simulink model "MicroFSMPCCLACPU1"  (R2024a)
settings: Solver=FixedStepAuto  StartTime=0.0  StopTime=Inf  RelTol=1e-3  EnableMultiTasking=on
values from neighbouring files (symbols this model uses):
  ar = single(round(1/10,3))    [Para_Motor_Micro.m]
  PI_params = mcb.internal.SetControllerParameters(pmsm,inverter,SI_System,T_pwm,Ts,Ts_speed)    [Para_Motor_Micro.m]
  Tabf = round(Tab',3)    [Para_Motor_Micro.m]
  target = mcb_SetProcessorDetails('F28379D',PWM_frequency)    [Para_Motor_Micro.m]
  Ts = T_pwm    (= 3e-05)    [Para_Motor_Micro.m]
  Ts_com = 2*1*Ts    (= 6e-05)    [Para_Motor_Micro.m]
undefined symbols (not defined in the file or in its folder): C28x, codertarget, CPU1, CPU2, Down, dyV, gmax, GPTRIP1SEL, GPTRIP2SEL, inverter, Ls, PWM_Counter_PeriodVel, R, Tab, Tv, Tvz, TZ1, TZ2, ud, Up
libraries: mcbcontrolslib x28, c2802xlib x18, c2837xDlib x13, dsparch4 x6, eeTransforms x5, slpidlib x4, mcbpositiondecoderlib x3, simulink x2, c2806xlib x1, spsabctoAlphaBetaZeroLib x1, c280xlib x1, c2000lib x1
(part 4 of 8)

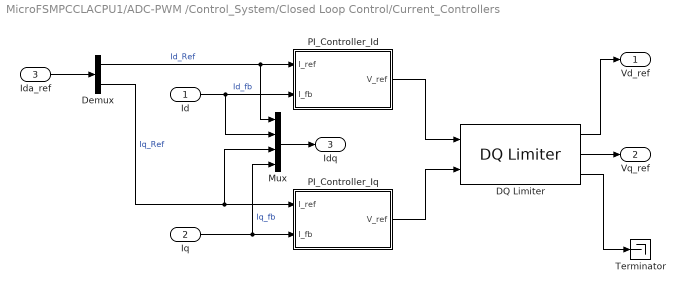
== system MicroFSMPCCLACPU1/ADC-PWM /Control_System/Closed Loop Control/Current_Controllers ==
  Id : Inport
  Iq : Inport  Port=2
  Ida_ref : Inport  Port=3
  DQ Limiter : mcbcontrolslib/DQ Limiter  satMethodInputType=Specify via dialog  satMethodSelected=D-Q equivalence  satLimitInputType=Specify via dialog  Vmax=inverter.V_dc/sqrt(3) *0.95
  Demux : Demux  Outputs=2
  Mux : Mux
  PI_Controller_Id : Subsystem
  PI_Controller_Iq : Subsystem
  Terminator : Terminator
  Vd_ref : Outport  VectorParamsAs1DForOutWhenUnconnected=off
  Vq_ref : Outport  Port=2  VectorParamsAs1DForOutWhenUnconnected=off
  Idq : Outport  Port=3  VectorParamsAs1DForOutWhenUnconnected=off
  wires:
  Iq/1 -> Mux/4, PI_Controller_Iq/2(I_fb)  "Iq_fb"
  Id/1 -> Mux/2, PI_Controller_Id/2(I_fb)  "Id_fb"
  Demux/1 -> Mux/1, PI_Controller_Id/1(I_ref)  "Id_Ref"
  Demux/2 -> Mux/3, PI_Controller_Iq/1(I_ref)  "Iq_Ref"
  Ida_ref/1 -> Demux/1
  Mux/1 -> Idq/1
  PI_Controller_Id/1(V_ref) -> DQ Limiter/1
  PI_Controller_Iq/1(V_ref) -> DQ Limiter/2
  DQ Limiter/2 -> Vq_ref/1
  DQ Limiter/1 -> Vd_ref/1
  DQ Limiter/3 -> Terminator/1

== system MicroFSMPCCLACPU1/ADC-PWM /Control_System/Closed Loop Control/Subsystem ==
  FCEM : Inport
  Demux5 : Demux  Outputs=2
  IIR Filter10 : mcbcontrolslib/IIR Filter  VariantControl=Low Pass Filter  VariantSelect=Low-pass  Filter_constant=0.2  advancedSettings=off  Ts=5e-5  cutOff_freq=795.7747
  IIR Filter9 : mcbcontrolslib/IIR Filter  VariantControl=Low Pass Filter  VariantSelect=Low-pass  Filter_constant=0.2  advancedSettings=off  Ts=5e-5  cutOff_freq=795.7747
  Mux7 : Mux  Inputs=2
  Out1 : Outport
  wires:
  IIR Filter9/1 -> Mux7/1
  Demux5/1 -> IIR Filter9/1
  Demux5/2 -> IIR Filter10/1
  IIR Filter10/1 -> Mux7/2
  Mux7/1 -> Out1/1
  FCEM/1 -> Demux5/1

== system MicroFSMPCCLACPU1/ADC-PWM /Mesurments/Position Mesurment/IndexFinder ==
  In1 : Inport
  Enable : EnablePort
  AND : Logic  AllPortsSameDT=off  OutDataTypeStr=boolean
  Compare To Constant : simulink/Logic and Bit Operations/Compare To Constant  relop===  const=0  OutDataTypeStr=boolean
  Compare To Constant1 : simulink/Logic and Bit Operations/Compare To Constant  relop=>  const=0  OutDataTypeStr=boolean
  Delay3 : Delay  DelayLength=1
  EnClosedLoop : Outport
  wires:
  In1/1 -> Delay3/1, Compare To Constant1/1
  Compare To Constant1/1 -> AND/2
  Compare To Constant/1 -> AND/1
  Delay3/1 -> Compare To Constant/1
  AND/1 -> EnClosedLoop/1

== system MicroFSMPCCLACPU1/ADC-PWM /Control_System/CLA Subsystem Current control/Current_Controllers/PI_Controller_Id ==
  I_ref : Inport
  I_fb : Inport  Port=2
  Data Store Read1 : DataStoreRead  DataStoreName=Enable  IndexOptions=Index vector (dialog)  Indices=1  OutputSizes=1
  Discrete PI Controller with anti-windup & reset : slpidlib/PID Controller  Controller=PI  Form=Parallel  TimeDomain=Discrete-time  UseExternalTs=off  SampleTime=-1  IntegratorMethod=Forward Euler  FilterMethod=Forward Euler  ControllerParametersSource=external  P=1  I=1  UseKiTs=on  D=0  N=100  UseFilter=on  TunerSelectOption=Transfer Function Based (PID Tuner App)  InitialConditionSource=external  InitialConditionForIntegrator=0  InitialConditionForFilter=0  DifferentiatorICPrevScaledInput=0  ExternalReset=level  TrackingMode=off  Kt=1  LimitOutput=on  SatLimitsSource=internal  UpperSaturationLimit=inverter.V_dc/sqrt(3)  LowerSaturationLimit=-inverter.V_dc/sqrt(3)  LinearizeAsGain=on  AntiWindupMode=clamping  Kb=1  LimitIntegrator=off  UpperIntegratorSaturationLimit=inf  LowerIntegratorSaturationLimit=-inf  RndMeth=Simplest  POutMin=[]  POutMax=[]  IOutMin=[]  IOutMax=[]  DOutMin=[]  DOutMax=[]  NOutMin=[]  NOutMax=[]  SumOutMin=[]  SumOutMax=[]  SaturationOutDataTypeStr=Inherit: Inherit via back propagation  SaturationOutMin=[]  SaturationOutMax=[]  PParamMin=[]  PParamMax=[]  IParamMin=[]  IParamMax=[]  DParamMin=[]  DParamMax=[]  NParamMin=[]  NParamMax=[]  KbParamMin=[]  KbParamMax=[]  KtParamMin=[]  KtParamMax=[]  KbOutMin=[]  KbOutMax=[]  KtOutMin=[]  KtOutMax=[]  IntegratorOutMin=[]  IntegratorOutMax=[]  FilterOutMin=[]  FilterOutMax=[]  SumI1OutMin=[]  SumI1OutMax=[]  SumI2OutMin=[]  SumI2OutMax=[]  SumI3OutMin=[]  SumI3OutMax=[]  SumI4OutMin=[]  SumI4OutMax=[]  SumDOutMin=[]  SumDOutMax=[]  DifferentiatorOutMin=[]  DifferentiatorOutMax=[]  FilterDiffOutCoefMin=[]  FilterDiffOutCoefMax=[]  ReciprocalOutMin=[]  ReciprocalOutMax=[]  SumDenOutMin=[]  SumDenOutMax=[]  SumNumOutMin=[]  SumNumOutMax=[]  DivideOutMin=[]  DivideOutMax=[]  UdiffTsProdOutMin=[]  UdiffTsProdOutMax=[]  NTsProdOutMin=[]  NTsProdOutMax=[]  UintegralTsProdOutMin=[]  UintegralTsProdOutMax=[]  UngainTsProdOutMin=[]  UngainTsProdOutMax=[]  ClampingZeroOutDataTypeStr=Inherit: Inherit via back propagation  ClampingZeroOutMin=[]  ClampingZeroOutMax=[]  FilterDenConstantOutDataTypeStr=Inherit: Inherit via back propagation  FilterDenConstantOutMin=[]  FilterDenConstantOutMax=[]  PCopyOutDataTypeStr=Inherit: Inherit via back propagation  PCopyOutMin=[]  PCopyOutMax=[]  NCopyOutDataTypeStr=Inherit: Inherit via back propagation  NCopyOutMin=[]  NCopyOutMax=[]  IntegratorContinuousStateAttributes=''  IntegratorStateMustResolveToSignalObject=off  IntegratorRTWStateStorageClass=Auto  FilterContinuousStateAttributes=''  FilterStateMustResolveToSignalObject=off  FilterRTWStateStorageClass=Auto  ParallelPVariant=ExternalParameters  IdealPVariant=Disabled  IVariant=ExternalParameters  DVariant=Disabled  IntegratorVariant=Discrete  SatVariant=Enabled  AWVariant=DiscClampingParallel  PCopyVariant=Disabled  TRVariant=Disabled  FdbkBlocksVariant=Forward  IdealPFdbkVariant=Disabled  SatFdbkVariant=Disabled  DerivativeFilterVariant=Disabled  NVariant=Disabled  NCopyVariant=Disabled_SignalSpec  FilterICVariant=Disabled  IntegratorICVariant=ExternalICs  ExternalResetVariant=ExternalReset  TRSumVariant=Passthrough  SumFdbkVariant=Disabled  SumVariant=Sum_PI  TsampFilterVariant=InternalTs  TsampNgainVariant=Passthrough  TsampIntegralVariant=Passthrough  ExternalSaturationOutDataTypeStr=Inherit: Same as second input
      settings: LibrarySourceBlock=mcbcontrolslib/PI Controller
  Ki1 : Constant  Value=0  OutDataTypeStr=dataType  SampleTime=-1
  Ki2 : Constant  Value=PI_params.Ki_i * Ts  OutDataTypeStr=dataType  SampleTime=-1
  Kp : Constant  Value=PI_params.Kp_i  OutDataTypeStr=dataType  SampleTime=-1
  Logical Operator : Logic  Operator=NOT  IconShape=distinctive  AllPortsSameDT=off  OutDataTypeStr=boolean
  Sum : Sum  Inputs=|+-  OutDataTypeStr=Inherit: Same as first input
  V_ref : Outport  VectorParamsAs1DForOutWhenUnconnected=off
  wires:
  I_ref/1 -> Sum/1
  I_fb/1 -> Sum/2
  Data Store Read1/1 -> Logical Operator/1
  Discrete PI Controller with anti-windup & reset/1 -> V_ref/1
  Sum/1 -> Discrete PI Controller with anti-windup & reset/1
  Logical Operator/1 -> Discrete PI Controller with anti-windup & reset/4
  Ki1/1 -> Discrete PI Controller with anti-windup & reset/5
  Kp/1 -> Discrete PI Controller with anti-windup & reset/2
  Ki2/1 -> Discrete PI Controller with anti-windup & reset/3

== system MicroFSMPCCLACPU1/ADC-PWM /Control_System/CLA Subsystem Current control/Current_Controllers/PI_Controller_Iq ==
  I_ref : Inport
  I_fb : Inport  Port=2
  Data Store Read1 : DataStoreRead  DataStoreName=Enable  IndexOptions=Index vector (dialog)  Indices=1  OutputSizes=1
  Discrete PI Controller with anti-windup & reset : slpidlib/PID Controller  Controller=PI  Form=Parallel  TimeDomain=Discrete-time  UseExternalTs=off  SampleTime=-1  IntegratorMethod=Forward Euler  FilterMethod=Forward Euler  ControllerParametersSource=external  P=1  I=1  UseKiTs=on  D=0  N=100  UseFilter=on  TunerSelectOption=Transfer Function Based (PID Tuner App)  InitialConditionSource=external  InitialConditionForIntegrator=0  InitialConditionForFilter=0  DifferentiatorICPrevScaledInput=0  ExternalReset=level  TrackingMode=off  Kt=1  LimitOutput=on  SatLimitsSource=internal  UpperSaturationLimit=inverter.V_dc/sqrt(3)  LowerSaturationLimit=-inverter.V_dc/sqrt(3)  LinearizeAsGain=on  AntiWindupMode=clamping  Kb=1  LimitIntegrator=off  UpperIntegratorSaturationLimit=inf  LowerIntegratorSaturationLimit=-inf  RndMeth=Simplest  POutMin=[]  POutMax=[]  IOutMin=[]  IOutMax=[]  DOutMin=[]  DOutMax=[]  NOutMin=[]  NOutMax=[]  SumOutMin=[]  SumOutMax=[]  SaturationOutDataTypeStr=Inherit: Inherit via back propagation  SaturationOutMin=[]  SaturationOutMax=[]  PParamMin=[]  PParamMax=[]  IParamMin=[]  IParamMax=[]  DParamMin=[]  DParamMax=[]  NParamMin=[]  NParamMax=[]  KbParamMin=[]  KbParamMax=[]  KtParamMin=[]  KtParamMax=[]  KbOutMin=[]  KbOutMax=[]  KtOutMin=[]  KtOutMax=[]  IntegratorOutMin=[]  IntegratorOutMax=[]  FilterOutMin=[]  FilterOutMax=[]  SumI1OutMin=[]  SumI1OutMax=[]  SumI2OutMin=[]  SumI2OutMax=[]  SumI3OutMin=[]  SumI3OutMax=[]  SumI4OutMin=[]  SumI4OutMax=[]  SumDOutMin=[]  SumDOutMax=[]  DifferentiatorOutMin=[]  DifferentiatorOutMax=[]  FilterDiffOutCoefMin=[]  FilterDiffOutCoefMax=[]  ReciprocalOutMin=[]  ReciprocalOutMax=[]  SumDenOutMin=[]  SumDenOutMax=[]  SumNumOutMin=[]  SumNumOutMax=[]  DivideOutMin=[]  DivideOutMax=[]  UdiffTsProdOutMin=[]  UdiffTsProdOutMax=[]  NTsProdOutMin=[]  NTsProdOutMax=[]  UintegralTsProdOutMin=[]  UintegralTsProdOutMax=[]  UngainTsProdOutMin=[]  UngainTsProdOutMax=[]  ClampingZeroOutDataTypeStr=Inherit: Inherit via back propagation  ClampingZeroOutMin=[]  ClampingZeroOutMax=[]  FilterDenConstantOutDataTypeStr=Inherit: Inherit via back propagation  FilterDenConstantOutMin=[]  FilterDenConstantOutMax=[]  PCopyOutDataTypeStr=Inherit: Inherit via back propagation  PCopyOutMin=[]  PCopyOutMax=[]  NCopyOutDataTypeStr=Inherit: Inherit via back propagation  NCopyOutMin=[]  NCopyOutMax=[]  IntegratorContinuousStateAttributes=''  IntegratorStateMustResolveToSignalObject=off  IntegratorRTWStateStorageClass=Auto  FilterContinuousStateAttributes=''  FilterStateMustResolveToSignalObject=off  FilterRTWStateStorageClass=Auto  ParallelPVariant=ExternalParameters  IdealPVariant=Disabled  IVariant=ExternalParameters  DVariant=Disabled  IntegratorVariant=Discrete  SatVariant=Enabled  AWVariant=DiscClampingParallel  PCopyVariant=Disabled  TRVariant=Disabled  FdbkBlocksVariant=Forward  IdealPFdbkVariant=Disabled  SatFdbkVariant=Disabled  DerivativeFilterVariant=Disabled  NVariant=Disabled  NCopyVariant=Disabled_SignalSpec  FilterICVariant=Disabled  IntegratorICVariant=ExternalICs  ExternalResetVariant=ExternalReset  TRSumVariant=Passthrough  SumFdbkVariant=Disabled  SumVariant=Sum_PI  TsampFilterVariant=InternalTs  TsampNgainVariant=Passthrough  TsampIntegralVariant=Passthrough  ExternalSaturationOutDataTypeStr=Inherit: Same as second input
      settings: LibrarySourceBlock=mcbcontrolslib/PI Controller
  Ki1 : Constant  Value=PI_params.Ki_i * Ts  OutDataTypeStr=dataType  SampleTime=-1
  Kp : Constant  Value=PI_params.Kp_i  OutDataTypeStr=dataType  SampleTime=-1
  Kp1 : Constant  Value=0  OutDataTypeStr=dataType  SampleTime=-1
  Logical Operator : Logic  Operator=NOT  IconShape=distinctive  AllPortsSameDT=off  OutDataTypeStr=boolean
  Sum : Sum  Inputs=|+-  OutDataTypeStr=Inherit: Same as first input
  V_ref : Outport  VectorParamsAs1DForOutWhenUnconnected=off
  wires:
  Discrete PI Controller with anti-windup & reset/1 -> V_ref/1
  Data Store Read1/1 -> Logical Operator/1
  I_fb/1 -> Sum/2
  I_ref/1 -> Sum/1
  Sum/1 -> Discrete PI Controller with anti-windup & reset/1
  Logical Operator/1 -> Discrete PI Controller with anti-windup & reset/4
  Kp1/1 -> Discrete PI Controller with anti-windup & reset/5
  Kp/1 -> Discrete PI Controller with anti-windup & reset/2
  Ki1/1 -> Discrete PI Controller with anti-windup & reset/3

== system MicroFSMPCCLACPU1/ADC-PWM /Control_System/Closed Loop Control/Current_Controllers/PI_Controller_Id ==
  I_ref : Inport
  I_fb : Inport  Port=2
  Data Store Read1 : DataStoreRead  DataStoreName=Enable  IndexOptions=Index vector (dialog)  Indices=1  OutputSizes=1
  Discrete PI Controller with anti-windup & reset : slpidlib/PID Controller  Controller=PI  Form=Parallel  TimeDomain=Discrete-time  UseExternalTs=off  SampleTime=-1  IntegratorMethod=Forward Euler  FilterMethod=Forward Euler  ControllerParametersSource=external  P=1  I=1  UseKiTs=on  D=0  N=100  UseFilter=on  TunerSelectOption=Transfer Function Based (PID Tuner App)  InitialConditionSource=external  InitialConditionForIntegrator=0  InitialConditionForFilter=0  DifferentiatorICPrevScaledInput=0  ExternalReset=level  TrackingMode=off  Kt=1  LimitOutput=on  SatLimitsSource=internal  UpperSaturationLimit=inverter.V_dc/sqrt(3)  LowerSaturationLimit=-inverter.V_dc/sqrt(3)  LinearizeAsGain=on  AntiWindupMode=clamping  Kb=1  LimitIntegrator=off  UpperIntegratorSaturationLimit=inf  LowerIntegratorSaturationLimit=-inf  RndMeth=Simplest  POutMin=[]  POutMax=[]  IOutMin=[]  IOutMax=[]  DOutMin=[]  DOutMax=[]  NOutMin=[]  NOutMax=[]  SumOutMin=[]  SumOutMax=[]  SaturationOutDataTypeStr=Inherit: Inherit via back propagation  SaturationOutMin=[]  SaturationOutMax=[]  PParamMin=[]  PParamMax=[]  IParamMin=[]  IParamMax=[]  DParamMin=[]  DParamMax=[]  NParamMin=[]  NParamMax=[]  KbParamMin=[]  KbParamMax=[]  KtParamMin=[]  KtParamMax=[]  KbOutMin=[]  KbOutMax=[]  KtOutMin=[]  KtOutMax=[]  IntegratorOutMin=[]  IntegratorOutMax=[]  FilterOutMin=[]  FilterOutMax=[]  SumI1OutMin=[]  SumI1OutMax=[]  SumI2OutMin=[]  SumI2OutMax=[]  SumI3OutMin=[]  SumI3OutMax=[]  SumI4OutMin=[]  SumI4OutMax=[]  SumDOutMin=[]  SumDOutMax=[]  DifferentiatorOutMin=[]  DifferentiatorOutMax=[]  FilterDiffOutCoefMin=[]  FilterDiffOutCoefMax=[]  ReciprocalOutMin=[]  ReciprocalOutMax=[]  SumDenOutMin=[]  SumDenOutMax=[]  SumNumOutMin=[]  SumNumOutMax=[]  DivideOutMin=[]  DivideOutMax=[]  UdiffTsProdOutMin=[]  UdiffTsProdOutMax=[]  NTsProdOutMin=[]  NTsProdOutMax=[]  UintegralTsProdOutMin=[]  UintegralTsProdOutMax=[]  UngainTsProdOutMin=[]  UngainTsProdOutMax=[]  ClampingZeroOutDataTypeStr=Inherit: Inherit via back propagation  ClampingZeroOutMin=[]  ClampingZeroOutMax=[]  FilterDenConstantOutDataTypeStr=Inherit: Inherit via back propagation  FilterDenConstantOutMin=[]  FilterDenConstantOutMax=[]  PCopyOutDataTypeStr=Inherit: Inherit via back propagation  PCopyOutMin=[]  PCopyOutMax=[]  NCopyOutDataTypeStr=Inherit: Inherit via back propagation  NCopyOutMin=[]  NCopyOutMax=[]  IntegratorContinuousStateAttributes=''  IntegratorStateMustResolveToSignalObject=off  IntegratorRTWStateStorageClass=Auto  FilterContinuousStateAttributes=''  FilterStateMustResolveToSignalObject=off  FilterRTWStateStorageClass=Auto  ParallelPVariant=ExternalParameters  IdealPVariant=Disabled  IVariant=ExternalParameters  DVariant=Disabled  IntegratorVariant=Discrete  SatVariant=Enabled  AWVariant=DiscClampingParallel  PCopyVariant=Disabled  TRVariant=Disabled  FdbkBlocksVariant=Forward  IdealPFdbkVariant=Disabled  SatFdbkVariant=Disabled  DerivativeFilterVariant=Disabled  NVariant=Disabled  NCopyVariant=Disabled_SignalSpec  FilterICVariant=Disabled  IntegratorICVariant=ExternalICs  ExternalResetVariant=ExternalReset  TRSumVariant=Passthrough  SumFdbkVariant=Disabled  SumVariant=Sum_PI  TsampFilterVariant=InternalTs  TsampNgainVariant=Passthrough  TsampIntegralVariant=Passthrough  ExternalSaturationOutDataTypeStr=Inherit: Same as second input
      settings: LibrarySourceBlock=mcbcontrolslib/PI Controller
  Ki1 : Constant  Value=0  OutDataTypeStr=dataType  SampleTime=-1
  Ki2 : Constant  Value=PI_params.Ki_i * Ts  OutDataTypeStr=dataType  SampleTime=-1
  Kp : Constant  Value=PI_params.Kp_i  OutDataTypeStr=dataType  SampleTime=-1
  Logical Operator : Logic  Operator=NOT  IconShape=distinctive  AllPortsSameDT=off  OutDataTypeStr=boolean
  Sum : Sum  Inputs=|+-  OutDataTypeStr=Inherit: Same as first input
  V_ref : Outport  VectorParamsAs1DForOutWhenUnconnected=off
  wires:
  I_ref/1 -> Sum/1
  I_fb/1 -> Sum/2
  Data Store Read1/1 -> Logical Operator/1
  Discrete PI Controller with anti-windup & reset/1 -> V_ref/1
  Sum/1 -> Discrete PI Controller with anti-windup & reset/1
  Logical Operator/1 -> Discrete PI Controller with anti-windup & reset/4
  Ki1/1 -> Discrete PI Controller with anti-windup & reset/5
  Kp/1 -> Discrete PI Controller with anti-windup & reset/2
  Ki2/1 -> Discrete PI Controller with anti-windup & reset/3

== system MicroFSMPCCLACPU1/ADC-PWM /Control_System/Closed Loop Control/Current_Controllers/PI_Controller_Iq ==
  I_ref : Inport
  I_fb : Inport  Port=2
  Data Store Read1 : DataStoreRead  DataStoreName=Enable  IndexOptions=Index vector (dialog)  Indices=1  OutputSizes=1
  Discrete PI Controller with anti-windup & reset : slpidlib/PID Controller  Controller=PI  Form=Parallel  TimeDomain=Discrete-time  UseExternalTs=off  SampleTime=-1  IntegratorMethod=Forward Euler  FilterMethod=Forward Euler  ControllerParametersSource=external  P=1  I=1  UseKiTs=on  D=0  N=100  UseFilter=on  TunerSelectOption=Transfer Function Based (PID Tuner App)  InitialConditionSource=external  InitialConditionForIntegrator=0  InitialConditionForFilter=0  DifferentiatorICPrevScaledInput=0  ExternalReset=level  TrackingMode=off  Kt=1  LimitOutput=on  SatLimitsSource=internal  UpperSaturationLimit=inverter.V_dc/sqrt(3)  LowerSaturationLimit=-inverter.V_dc/sqrt(3)  LinearizeAsGain=on  AntiWindupMode=clamping  Kb=1  LimitIntegrator=off  UpperIntegratorSaturationLimit=inf  LowerIntegratorSaturationLimit=-inf  RndMeth=Simplest  POutMin=[]  POutMax=[]  IOutMin=[]  IOutMax=[]  DOutMin=[]  DOutMax=[]  NOutMin=[]  NOutMax=[]  SumOutMin=[]  SumOutMax=[]  SaturationOutDataTypeStr=Inherit: Inherit via back propagation  SaturationOutMin=[]  SaturationOutMax=[]  PParamMin=[]  PParamMax=[]  IParamMin=[]  IParamMax=[]  DParamMin=[]  DParamMax=[]  NParamMin=[]  NParamMax=[]  KbParamMin=[]  KbParamMax=[]  KtParamMin=[]  KtParamMax=[]  KbOutMin=[]  KbOutMax=[]  KtOutMin=[]  KtOutMax=[]  IntegratorOutMin=[]  IntegratorOutMax=[]  FilterOutMin=[]  FilterOutMax=[]  SumI1OutMin=[]  SumI1OutMax=[]  SumI2OutMin=[]  SumI2OutMax=[]  SumI3OutMin=[]  SumI3OutMax=[]  SumI4OutMin=[]  SumI4OutMax=[]  SumDOutMin=[]  SumDOutMax=[]  DifferentiatorOutMin=[]  DifferentiatorOutMax=[]  FilterDiffOutCoefMin=[]  FilterDiffOutCoefMax=[]  ReciprocalOutMin=[]  ReciprocalOutMax=[]  SumDenOutMin=[]  SumDenOutMax=[]  SumNumOutMin=[]  SumNumOutMax=[]  DivideOutMin=[]  DivideOutMax=[]  UdiffTsProdOutMin=[]  UdiffTsProdOutMax=[]  NTsProdOutMin=[]  NTsProdOutMax=[]  UintegralTsProdOutMin=[]  UintegralTsProdOutMax=[]  UngainTsProdOutMin=[]  UngainTsProdOutMax=[]  ClampingZeroOutDataTypeStr=Inherit: Inherit via back propagation  ClampingZeroOutMin=[]  ClampingZeroOutMax=[]  FilterDenConstantOutDataTypeStr=Inherit: Inherit via back propagation  FilterDenConstantOutMin=[]  FilterDenConstantOutMax=[]  PCopyOutDataTypeStr=Inherit: Inherit via back propagation  PCopyOutMin=[]  PCopyOutMax=[]  NCopyOutDataTypeStr=Inherit: Inherit via back propagation  NCopyOutMin=[]  NCopyOutMax=[]  IntegratorContinuousStateAttributes=''  IntegratorStateMustResolveToSignalObject=off  IntegratorRTWStateStorageClass=Auto  FilterContinuousStateAttributes=''  FilterStateMustResolveToSignalObject=off  FilterRTWStateStorageClass=Auto  ParallelPVariant=ExternalParameters  IdealPVariant=Disabled  IVariant=ExternalParameters  DVariant=Disabled  IntegratorVariant=Discrete  SatVariant=Enabled  AWVariant=DiscClampingParallel  PCopyVariant=Disabled  TRVariant=Disabled  FdbkBlocksVariant=Forward  IdealPFdbkVariant=Disabled  SatFdbkVariant=Disabled  DerivativeFilterVariant=Disabled  NVariant=Disabled  NCopyVariant=Disabled_SignalSpec  FilterICVariant=Disabled  IntegratorICVariant=ExternalICs  ExternalResetVariant=ExternalReset  TRSumVariant=Passthrough  SumFdbkVariant=Disabled  SumVariant=Sum_PI  TsampFilterVariant=InternalTs  TsampNgainVariant=Passthrough  TsampIntegralVariant=Passthrough  ExternalSaturationOutDataTypeStr=Inherit: Same as second input
      settings: LibrarySourceBlock=mcbcontrolslib/PI Controller
  Ki1 : Constant  Value=PI_params.Ki_i * Ts  OutDataTypeStr=dataType  SampleTime=-1
  Kp : Constant  Value=PI_params.Kp_i  OutDataTypeStr=dataType  SampleTime=-1
  Kp1 : Constant  Value=0  OutDataTypeStr=dataType  SampleTime=-1
  Logical Operator : Logic  Operator=NOT  IconShape=distinctive  AllPortsSameDT=off  OutDataTypeStr=boolean
  Sum : Sum  Inputs=|+-  OutDataTypeStr=Inherit: Same as first input
  V_ref : Outport  VectorParamsAs1DForOutWhenUnconnected=off
  wires:
  Discrete PI Controller with anti-windup & reset/1 -> V_ref/1
  Data Store Read1/1 -> Logical Operator/1
  I_fb/1 -> Sum/2
  I_ref/1 -> Sum/1
  Sum/1 -> Discrete PI Controller with anti-windup & reset/1
  Logical Operator/1 -> Discrete PI Controller with anti-windup & reset/4
  Kp1/1 -> Discrete PI Controller with anti-windup & reset/5
  Kp/1 -> Discrete PI Controller with anti-windup & reset/2
  Ki1/1 -> Discrete PI Controller with anti-windup & reset/3

== matlab function MicroFSMPCCLACPU1/ADC-PWM /Control_System/CLA Subsystem Current control/TESTCLA ==
  settings: updateMethod=DISCRETE
  data: I input; Gate output size=3; FEM input size=2; moder input single

function Gate       = fcn(I,FEM,moder)
TA=single(0);
TB=single(0);
TC=single(0);
%  persistent    Gates
%      if isempty(Gates)
%         Gates=single([0,0,0]');
%  
%        end

%%%%%%Read mesurments%%%%%%%%%%%%
iA=I(1);
iB=I(2);
eA=FEM(1);
eB=FEM(2);

Ta=single(0.1*0.25);
Tb=single(0.1*0);

TA=single((moder==1)*(Tb+Ta)+(moder==6)*(Tb+Ta)+(moder==2)*(Ta)+(moder==5)*(Tb));
TB=single((moder==1)*(Tb)+(moder==2)*(Tb+Ta)+(moder==3)*(Tb+Ta)+(moder==4)*(Ta));
TC=single((moder==6)*(Ta)+(moder==3)*(Tb)+(moder==4)*(Tb+Ta)+(moder==5)*(Tb+Ta));
  
% TA=single(0.1*moder);
% TB=single(0.1);
% TC=single(0.1);
%%%Optimized modulation.
% if moder==1
% TA=single(Tb+Ta);
% TB=single(Tb);
% TC=single(0);
% elseif moder==2
% TA=single(Ta);
% TB=single(Tb+Ta);
% TC=single(0);
% elseif moder==3
% TA=single(0);
% TB=single(Tb+Ta);
% TC=single(Tb);   
% elseif moder==4
% TA=single(0);
% TB=single(Ta);
% TC=single(Tb+Ta); 
% elseif moder==5
% TA=single(Tb);
% TB=single(0);
% TC=single(Tb+Ta); 
% elseif moder==6
% TA=single(Tb+Ta);
% TB=single(0);
% TC=single(Ta); 
% else
% TA=single(0);
% TB=single(0);
% TC=single(0);   
% end



Gates=[TA,TB,TC]';
Gate=Gates;

== matlab function MicroFSMPCCLACPU1/ADC-PWM /Control_System/CLA Subsystem Current control/FS-MPC opt tiempo complex Clean CLA ==
  settings: updateMethod=DISCRETE
  data: I input single size=2; Gate output single size=3; FEM input single size=2; iAref input single size=1; iBref input single size=1; mode input single size=1; ud input

function Gate       = fcn(I,FEM,iAref,iBref,mode,ud)


%%%%%Init Parameters%%%%%%%
% 
Ts=single(3e-5);
R=single(1) ;
Ls=single(0.002871);
%ud=single(170);
gmax=single(1000);
n=single(11);
moder=mode;
%Tabfn=single([0,0;0,0;0,0;0,0]);
p1=single(0);
p2=single(0);

 persistent     Gates Gop jop  Tr Tao Tbo  
  if isempty(Gates)
        Gates=single([0,0,0]');
        Gop=gmax;
        jop=single(1);
        Tr=single(0);
        Tao=single(0);
Tbo=single(0);

     end


% ar=single(0.9*0.143);
% Tabf=single(0.9*[0.286	0;
% 0	0.286;
% 0.572	0;
% 0	0.572;
% 0.858	0;
% 0	0.858;
% 1	0;
% 0	1;
% 1	0;
% 0	1;
% 0	0;]);

ar=single(0.129);

Tabf=single([0.242	0;
0	0.242;
0.484	0;
0	0.484;
0.726	0;
0	0.726;
1	0;
0	1;
1	0;
0	1;
0	0;]);


%%%%%%Read mesurments%%%%%%%%%%%%
iA=I(1);
iB=I(2);
eA=-FEM(1);
eB=-FEM(2);




% % %%%7 Vectores totales
 if mode==1
 u1=ud*[2/3	,	0	;
1/3	,	1/sqrt(3);
0	,	0	;];
elseif mode==2
 u1=ud*[1/3	,	1/sqrt(3)	;
-1/3	,	1/sqrt(3)	;
0	,	0	;];   
elseif mode==3
 u1=ud*[-1/3	,	1/sqrt(3)	;
-2/3	,	0	;
0	,	0	;];  
 elseif mode==4
 u1=ud*[-2/3	,	0	;
-1/3	,	-1/sqrt(3)	;
0	,	0	;];
 elseif mode==5
 u1=ud*[-1/3	,	-1/sqrt(3)	;
1/3	,	-1/sqrt(3)	;
0	,	0	;];
 elseif mode==6
 u1=ud*[1/3	,	-1/sqrt(3)	;
2/3	,	0	;
0	,	0	;];
else
 u1=ud*[2/3	,	0	;
1/3	,	1/sqrt(3);
0	,	0	;]; 
end
%%%%%%%




%%%%%%%%FSMPC%%%%%%%%%%%%%%%%%%%%%%%%%%%%%%%%%%%%%

      Gop=gmax;
      jop=single(1);
     %  ar=single(0.9/7);
%%%%%%For n loop N1  %%%%%% 





     uA1=u1(1,1);
     uB1=u1(1,2);
     uA2=u1(2,1);
     uB2=u1(2,2);

%%%%%%For n loop  %%%%%% 
     for j= 1:n    
   
if j==7
p1=Tr+ar;
p2=Tr-ar;
end

   if j<=n-5      
    T1=Tabf(j,1);
    T2=Tabf(j,2);
   elseif j<=n-3  
    T1=p1*Tabf(j,1);
    T2=p1*Tabf(j,2);
   else
    T1=p2*Tabf(j,1);
    T2=p2*Tabf(j,2);
   end


   uA=(T1*uA1 + T2*uA2);
   uB=(T1*uB1 + T2*uB2);
     
%%%%%%For loop %%%%%%%%%%%%%%%%%%%%%%%%%%%%%%%%% 
     iA1= iA + (1/Ls)*(Ts*uA)- (Ts/Ls)*(eA+R*iA);
     iB1=iB + (1/Ls)*(Ts*uB)- (Ts/Ls)*(eB+R*iB);

     G=(iAref-iA1)^2+(iBref-iB1)^2 ; 
     % G=abs(iAref-iA1)+abs(iBref-iB1) ; 
          if G<Gop
          Gop=G;
          %jop=j;
          Tr=T1+T2;
          Tao=T1;
          Tbo=T2;
          end
     end
%end
%%%%%%%%%%%%%%%%%%%%%%%%%%%%%%%%%%%%%%%%%%%%%%%%%
    
%%%%Apply conmutation states%%%%%%%%%%%%%%%%%%%%%%%  


Ta=Tao;
Tb=Tbo;
% To=single(1-Ta-Tb-0.1);

TA=(moder==1)*(Tb+Ta)+(moder==6)*(Tb+Ta)+(moder==2)*(Ta)+(moder==5)*(Tb);
TB=(moder==1)*(Tb)+(moder==2)*(Tb+Ta)+(moder==3)*(Tb+Ta)+(moder==4)*(Ta);
TC=(moder==6)*(Ta)+(moder==3)*(Tb)+(moder==4)*(Tb+Ta)+(moder==5)*(Tb+Ta);

% TA=(mode==1)*(To+Tb+Ta)+(mode==6)*(To+Tb+Ta)+(mode==2)*(To+Ta)+(mode==3)*(To)+(mode==4)*(To)+(mode==5)*(To+Tb);
% TB=(mode==6)*(To)+(mode==1)*(To+Tb)+(mode==2)*(To+Tb+Ta)+(mode==3)*(To+Tb+Ta)+(mode==4)*(To+Ta)+(mode==5)*(To);
% TC=(mode==6)*(To+Ta)+(mode==1)*(To)+(mode==2)*(To)+(mode==3)*(To+Tb)+(mode==4)*(To+Tb+Ta)+(mode==5)*(To+Tb+Ta);

Gates=[TA,TB,TC]';
%J=jop;
Gate=Gates;

== matlab function MicroFSMPCCLACPU1/ADC-PWM /Control_System/CLA Subsystem Current control/FS-MPC 2 Vectores solos modulado CLA1 ==
  settings: updateMethod=DISCRETE
  data: I input; Gate output size=3; FEM input size=2; iAref input; iBref input; mode input; ud input

function Gate        = fcn(I,FEM,iAref,iBref,mode,ud)
%function Gate       = fcn(I,FEM,iAref,iBref,mode,Ts, R, Ls, ud, gmax,dyV, Tab)


%%%%%Init Parameters%%%%%%%

Ts=single(4e-5);
R=single(1.1) ;
%Ls=single(0.002871);
Ls=single(0.00372);%%Mediciones
%ud=single(170);
gmax=single(1000);
n=single(15);

% Div=single(4); %%%%Numero de divisiones 
% dy0=single(0.12);
dyV=single(0.85);



%Tp=single(Ts*0.9);
 persistent    Gop jop Gates 
     if isempty(Gates)
        Gates=single([0,0,0]');
        Gop=gmax;
        jop=single(1);
  
     end


%%%%%%Read mesurments%%%%%%%%%%%%
iA=I(1);
iB=I(2);
eA=-FEM(1);
eB=-FEM(2);
moder=mode;

% % 
% % indexv=[1,1,1,1,1,1,1,1,1,1,2,2,2,2,3;
% %         1,1,1,1,1,1,2,2,2,3,2,2,2,3,3;
% %         1,1,1,2,2,3,2,2,3,3,2,2,3,3,3;
% %         1,2,3,2,3,3,2,3,3,3,2,3,3,3,3;];

Tab=single([0.143	0;
0	0.143;
0.286	0;
0	0.286;
0.429	0;
0	0.429;
0.572	0;
0	0.572;
0.715	0;
0	0.715;
0.858	0;
0	0.858;
1	0;
0	1;
0	0]);

if mode==1
   u1=ud*single([0	,	0	;
2/3	,	0	;
1/3	,	1/sqrt(3)]);
elseif mode==2
   u1=ud*single([0	,	0	;
1/3	,	1/sqrt(3)	;
-1/3	,	1/sqrt(3)	;]);   
elseif mode==3
   u1=ud*single([0	,	0	;
-1/3	,	1/sqrt(3)	;
-2/3	,	0	;]);  
 elseif mode==4
   u1=ud*single([0	,	0	;
-2/3	,	0	;
-1/3	,	-1/sqrt(3)	;]);
 elseif mode==5
   u1=ud*single([0	,	0	;
-1/3	,	-1/sqrt(3)	;
1/3	,	-1/sqrt(3)	;]);
 elseif mode==6
  u1=ud*single([0	,	0	;
1/3	,	-1/sqrt(3)	;
2/3	,	0	;]);
else
  u1=ud*single([0	,	0	;
2/3	,	0	;
1/3	,	1/sqrt(3)]); 
end

%%%%%%%%FSMPC%%%%%%%%%%%%%%%%%%%%%%%%%%%%%%%%%%%%%

     Gop=gmax;
     jop=single(1);
     uA1=u1(2,1);
     uB1=u1(2,2);
     uA2=u1(3,1);
     uB2=u1(3,2);

%%%%%%For n loop  %%%%%% 
     for j= 1:n    
   
    T1=Tab(j,1);
    T2=Tab(j,2);
    uA=dyV*(T1*uA1 + T2*uA2);%+dy0*uAnull;
    uB=dyV*(T1*uB1 + T2*uB2);%+dy0*uAnull;

%%%%%%For loop 3 combinacion de vectores%%%%%% 

     iA1= iA + (1/Ls)*(Ts*uA)- (Ts/Ls)*(eA+R*iA);
     iB1=iB + (1/Ls)*(Ts*uB)- (Ts/Ls)*(eB+R*iB);
     
     G=(iAref-iA1)^2+(iBref-iB1)^2 ; 

          if G<Gop
          Gop=G;
          jop=j;
          
          end
     end
%%%%Apply conmutation states%%%%%%%%%%%%%%%%%%%%%%%  
Ta=dyV*Tab(jop,1);
Tb=dyV*Tab(jop,2);
To=1-Ta-Tb-0.15;

% TA=(moder==1)*(Tb+Ta)+(moder==6)*(Tb+Ta)+(moder==2)*(Ta)+(moder==5)*(Tb);
% TB=(moder==1)*(Tb)+(moder==2)*(Tb+Ta)+(moder==3)*(Tb+Ta)+(moder==4)*(Ta);
% TC=(moder==6)*(Ta)+(moder==3)*(Tb)+(moder==4)*(Tb+Ta)+(moder==5)*(Tb+Ta);

TA=(mode==1)*(To+Tb+Ta)+(mode==6)*(To+Tb+Ta)+(mode==2)*(To+Ta)+(mode==3)*(To)+(mode==4)*(To)+(mode==5)*(To+Tb);
TB=(mode==6)*(To)+(mode==1)*(To+Tb)+(mode==2)*(To+Tb+Ta)+(mode==3)*(To+Tb+Ta)+(mode==4)*(To+Ta)+(mode==5)*(To);
TC=(mode==6)*(To+Ta)+(mode==1)*(To)+(mode==2)*(To)+(mode==3)*(To+Tb)+(mode==4)*(To+Tb+Ta)+(mode==5)*(To+Tb+Ta);
  

Gates=[TA,TB,TC]';
Gate=Gates;
%jo=jop;

== matlab function MicroFSMPCCLACPU1/ADC-PWM /Control_System/CLA Subsystem Current control/FS-MPC Simple CLA Mod ==
  settings: updateMethod=DISCRETE
  data: I input; Gate output size=3; FEM input; iAref input; iBref input; mode input; ud input

function Gate       = fcn(I,FEM,iAref,iBref,mode,ud)
%function [Gate,J,Vpred,Ipred]      = fcn(I,FEM,iAref,iBref,Vbus,mode)


%%%%%Init Parameters%%%%%%%
Ts=single(3e-5);
R=single(1.1) ;
%Ls=single(0.002871);
Ls=single(0.00372);%%Mediciones
ud=single(170);
gmax=single(1000);

n=single(3);
Tp=single(Ts*0.85);

 persistent    Gop jop Gates  %status1 %tick status1 
     if isempty(Gates)
        Gates=single([0,0,0]');
        Gop=gmax;
        jop=single(1);
     end


%%%%%%Read mesurments%%%%%%%%%%%%
iA=I(1);
iB=I(2);
eA=-FEM(1);
eB=-FEM(2);
moder=mode;

%%%% 7 vectors
%  status1=single([0,0,0;
%  1,0,0;
%  1,1,0; 
%  0,1,0;
%  0,1,1;
%  0,0,1;
%  1,0,1;]);   
%  u1=ud*single([0	,	0	;
%  2/3	,	0	;
%  1/3	,	1/sqrt(3);
% -1/3	,	1/sqrt(3);
% -2/3	,	0;
% -1/3	,	-1/sqrt(3);
%  1/3	,	-1/sqrt(3)	;]);
%%%%%%%


%%%%% Como en sim 
 if mode==1

 u1=ud*single([0	,	0	;
2/3	,	0	;
1/3	,	1/sqrt(3)]);
elseif mode==2

 u1=ud*single([0	,	0	;
1/3	,	1/sqrt(3)	;
-1/3	,	1/sqrt(3)	;]);   
elseif mode==3

 u1=ud*single([0	,	0	;
-1/3	,	1/sqrt(3)	;
-2/3	,	0	;]);  
 elseif mode==4

 u1=ud*single([0	,	0	;
-2/3	,	0	;
-1/3	,	-1/sqrt(3)	;]);
 elseif mode==5

 u1=ud*single([0	,	0	;
-1/3	,	-1/sqrt(3)	;
1/3	,	-1/sqrt(3)	;]);
 elseif mode==6

 u1=ud*single([0	,	0	;
1/3	,	-1/sqrt(3)	;
2/3	,	0	;]);

else

 u1=ud*single([0	,	0	;
2/3	,	0	;
1/3	,	1/sqrt(3)]); 
end






%%%%%%%%FSMPC%%%%%%%%%%%%%%%%%%%%%%%%%%%%%%%%%%%%%

     Gop=gmax;

%%%%%%For n loop  %%%%%% 
     for j= 1:n    
     uA1=u1(j,1);
     uB1=u1(j,2);


     iA1= iA + (1/Ls)*(Tp*uA1)- (Ts/Ls)*(eA+R*iA);
     iB1=iB + (1/Ls)*(Tp*uB1)- (Ts/Ls)*(eB+R*iB);
     
    
     G=(iAref-iA1)^2+(iBref-iB1)^2;%+ b*Z ; 

          if G<Gop
          Gop=G;
          jop=j;
          end
     end




Ta=single(0.85)*(jop==2);
Tb=single(0.85)*(jop==3);
% 
TA=(moder==1)*(Tb+Ta)+(moder==6)*(Tb+Ta)+(moder==2)*(Ta)+(moder==5)*(Tb);
TB=(moder==1)*(Tb)+(moder==2)*(Tb+Ta)+(moder==3)*(Tb+Ta)+(moder==4)*(Ta);
TC=(moder==6)*(Ta)+(moder==3)*(Tb)+(moder==4)*(Tb+Ta)+(moder==5)*(Tb+Ta);

% TA=(mode==1)*(To+Tb+Ta)+(mode==6)*(To+Tb+Ta)+(mode==2)*(To+Ta)+(mode==3)*(To)+(mode==4)*(To)+(mode==5)*(To+Tb);
% TB=(mode==6)*(To)+(mode==1)*(To+Tb)+(mode==2)*(To+Tb+Ta)+(mode==3)*(To+Tb+Ta)+(mode==4)*(To+Ta)+(mode==5)*(To);
% TC=(mode==6)*(To+Ta)+(mode==1)*(To)+(mode==2)*(To)+(mode==3)*(To+Tb)+(mode==4)*(To+Tb+Ta)+(mode==5)*(To+Tb+Ta);
  

%Gates=single(0.85*status1(jop,:)');
Gates=[TA,TB,TC]';
Gate=Gates;

== matlab function MicroFSMPCCLACPU1/ADC-PWM /Control_System/CLA Subsystem Current control/FS-MPC2_CLA(10) ==
  settings: updateMethod=DISCRETE
  data: I input; Gate output size=3; FEM input size=2; iAref input; iBref input; mode input; jo output

function [Gate,jo]       = fcn(I,FEM,iAref,iBref,mode)
%function Gate       = fcn(I,FEM,iAref,iBref,mode,Ts, R, Ls, ud, gmax,dyV, Tab)


%%%%%Init Parameters%%%%%%%

Ts=single(3e-5);
R=single(1.1) ;
Ls=single(0.00372);
ud=single(170);
gmax=single(1000);
n=single(10);

% Div=single(4); %%%%Numero de divisiones 
% dy0=single(0.12);
dyV=single(0.85);


%Tp=single(Ts*0.9);
 persistent    Gop jop Gates 
     if isempty(Gates)
        Gates=single([0,0,0]');
        Gop=gmax;
        jop=single(1);
  
     end


%%%%%%Read mesurments%%%%%%%%%%%%
iA=I(1);
iB=I(2);
eA=-FEM(1);
eB=-FEM(2);
moder=mode;



Tab=single([0         0;
    0.3330         0;
    0.6670         0;
    1.0000         0;
         0    0.3330;
    0.3330    0.3330;
    0.6670    0.3330;
         0    0.6670;
    0.3330    0.6670;
         0    1.0000]);

if mode==1
   u1=ud*single([0	,	0	;
2/3	,	0	;
1/3	,	1/sqrt(3)]);
elseif mode==2
   u1=ud*single([0	,	0	;
1/3	,	1/sqrt(3)	;
-1/3	,	1/sqrt(3)	;]);   
elseif mode==3
   u1=ud*single([0	,	0	;
-1/3	,	1/sqrt(3)	;
-2/3	,	0	;]);  
 elseif mode==4
   u1=ud*single([0	,	0	;
-2/3	,	0	;
-1/3	,	-1/sqrt(3)	;]);
 elseif mode==5
   u1=ud*single([0	,	0	;
-1/3	,	-1/sqrt(3)	;
1/3	,	-1/sqrt(3)	;]);
 elseif mode==6
  u1=ud*single([0	,	0	;
1/3	,	-1/sqrt(3)	;
2/3	,	0	;]);
else
  u1=ud*single([0	,	0	;
2/3	,	0	;
1/3	,	1/sqrt(3)]); 
end

%%%%%%%%FSMPC%%%%%%%%%%%%%%%%%%%%%%%%%%%%%%%%%%%%%

     Gop=gmax;
     jop=single(1);
     uA1=u1(2,1);
     uB1=u1(2,2);
     uA2=u1(3,1);
     uB2=u1(3,2);

%%%%%%For n loop  %%%%%% 
     for j= 1:n    
   
    T1=Tab(j,1);
    T2=Tab(j,2);
    uA=dyV*(T1*uA1 + T2*uA2);%+dy0*uAnull;
    uB=dyV*(T1*uB1 + T2*uB2);%+dy0*uAnull;

%%%%%%For loop 3 combinacion de vectores%%%%%% 

     iA1= iA + (1/Ls)*(Ts*uA)- (Ts/Ls)*(eA+R*iA);
     iB1=iB + (1/Ls)*(Ts*uB)- (Ts/Ls)*(eB+R*iB);
     
     G=(iAref-iA1)^2+(iBref-iB1)^2 ; 

          if G<Gop
          Gop=G;
          jop=j;
          
          end
     end
%%%%Apply conmutation states%%%%%%%%%%%%%%%%%%%%%%%  
Ta=dyV*Tab(jop,1);
Tb=dyV*Tab(jop,2);
To=single(1)-Ta-Tb-single(0.15);

% TA=(moder==1)*(Tb+Ta)+(moder==6)*(Tb+Ta)+(moder==2)*(Ta)+(moder==5)*(Tb);
% TB=(moder==1)*(Tb)+(moder==2)*(Tb+Ta)+(moder==3)*(Tb+Ta)+(moder==4)*(Ta);
% TC=(moder==6)*(Ta)+(moder==3)*(Tb)+(moder==4)*(Tb+Ta)+(moder==5)*(Tb+Ta);

TA=(mode==1)*(To+Tb+Ta)+(mode==6)*(To+Tb+Ta)+(mode==2)*(To+Ta)+(mode==3)*(To)+(mode==4)*(To)+(mode==5)*(To+Tb);
TB=(mode==6)*(To)+(mode==1)*(To+Tb)+(mode==2)*(To+Tb+Ta)+(mode==3)*(To+Tb+Ta)+(mode==4)*(To+Ta)+(mode==5)*(To);
TC=(mode==6)*(To+Ta)+(mode==1)*(To)+(mode==2)*(To)+(mode==3)*(To+Tb)+(mode==4)*(To+Tb+Ta)+(mode==5)*(To+Tb+Ta);


Gates=[TA,TB,TC]';
Gate=Gates;
jo=jop;

== matlab function MicroFSMPCCLACPU1/ADC-PWM /Control_System/CLA Subsystem Current control/FS-MPC2_CLA(21) ==
  settings: updateMethod=DISCRETE
  data: I input; Gate output size=3; FEM input size=2; iAref input; iBref input; mode input; jo output

function [Gate,jo]       = fcn(I,FEM,iAref,iBref,mode)
%function Gate       = fcn(I,FEM,iAref,iBref,mode,Ts, R, Ls, ud, gmax,dyV, Tab)


%%%%%Init Parameters%%%%%%%

Ts=single(3e-5);
R=single(1.1) ;
Ls=single(0.00372);
ud=single(170);
gmax=single(1000);
n=single(21);

% Div=single(4); %%%%Numero de divisiones 
% dy0=single(0.12);
dyV=single(0.85);


%Tp=single(Ts*0.9);
 persistent    Gop jop Gates 
     if isempty(Gates)
        Gates=single([0,0,0]');
        Gop=gmax;
        jop=single(1);
  
     end


%%%%%%Read mesurments%%%%%%%%%%%%
iA=I(1);
iB=I(2);
eA=-FEM(1);
eB=-FEM(2);
moder=mode;



Tab=single([0         0;
    0.2000         0;
    0.4000         0;
    0.6000         0;
    0.8000         0;
    1.0000         0;
         0    0.2000;
    0.2000    0.2000;
    0.4000    0.2000;
    0.6000    0.2000;
    0.8000    0.2000;
         0    0.4000;
    0.2000    0.4000;
    0.4000    0.4000;
    0.6000    0.4000;
         0    0.6000;
    0.2000    0.6000;
    0.4000    0.6000;
         0    0.8000;
    0.2000    0.8000;
         0    1.0000]);

if mode==1
   u1=ud*single([0	,	0	;
2/3	,	0	;
1/3	,	1/sqrt(3)]);
elseif mode==2
   u1=ud*single([0	,	0	;
1/3	,	1/sqrt(3)	;
-1/3	,	1/sqrt(3)	;]);   
elseif mode==3
   u1=ud*single([0	,	0	;
-1/3	,	1/sqrt(3)	;
-2/3	,	0	;]);  
 elseif mode==4
   u1=ud*single([0	,	0	;
-2/3	,	0	;
-1/3	,	-1/sqrt(3)	;]);
 elseif mode==5
   u1=ud*single([0	,	0	;
-1/3	,	-1/sqrt(3)	;
1/3	,	-1/sqrt(3)	;]);
 elseif mode==6
  u1=ud*single([0	,	0	;
1/3	,	-1/sqrt(3)	;
2/3	,	0	;]);
else
  u1=ud*single([0	,	0	;
2/3	,	0	;
1/3	,	1/sqrt(3)]); 
end

%%%%%%%%FSMPC%%%%%%%%%%%%%%%%%%%%%%%%%%%%%%%%%%%%%

     Gop=gmax;
     jop=single(1);
     uA1=u1(2,1);
     uB1=u1(2,2);
     uA2=u1(3,1);
     uB2=u1(3,2);

%%%%%%For n loop  %%%%%% 
     for j= 1:n    
   
    T1=Tab(j,1);
    T2=Tab(j,2);
    uA=dyV*(T1*uA1 + T2*uA2);%+dy0*uAnull;
    uB=dyV*(T1*uB1 + T2*uB2);%+dy0*uAnull;

%%%%%%For loop 3 combinacion de vectores%%%%%% 

     iA1= iA + (1/Ls)*(Ts*uA)- (Ts/Ls)*(eA+R*iA);
     iB1=iB + (1/Ls)*(Ts*uB)- (Ts/Ls)*(eB+R*iB);
     
     G=(iAref-iA1)^2+(iBref-iB1)^2 ; 

          if G<Gop
          Gop=G;
          jop=j;
          
          end
     end
%%%%Apply conmutation states%%%%%%%%%%%%%%%%%%%%%%%  
Ta=dyV*Tab(jop,1);
Tb=dyV*Tab(jop,2);
To=single(1)-Ta-Tb-single(0.15);

% TA=(moder==1)*(Tb+Ta)+(moder==6)*(Tb+Ta)+(moder==2)*(Ta)+(moder==5)*(Tb);
% TB=(moder==1)*(Tb)+(moder==2)*(Tb+Ta)+(moder==3)*(Tb+Ta)+(moder==4)*(Ta);
% TC=(moder==6)*(Ta)+(moder==3)*(Tb)+(moder==4)*(Tb+Ta)+(moder==5)*(Tb+Ta);

TA=(mode==1)*(To+Tb+Ta)+(mode==6)*(To+Tb+Ta)+(mode==2)*(To+Ta)+(mode==3)*(To)+(mode==4)*(To)+(mode==5)*(To+Tb);
TB=(mode==6)*(To)+(mode==1)*(To+Tb)+(mode==2)*(To+Tb+Ta)+(mode==3)*(To+Tb+Ta)+(mode==4)*(To+Ta)+(mode==5)*(To);
TC=(mode==6)*(To+Ta)+(mode==1)*(To)+(mode==2)*(To)+(mode==3)*(To+Tb)+(mode==4)*(To+Tb+Ta)+(mode==5)*(To+Tb+Ta);


Gates=[TA,TB,TC]';
Gate=Gates;
jo=jop;

== matlab function MicroFSMPCCLACPU1/ADC-PWM /Control_System/CLA Subsystem Current control/FS-MPC1_ CLA 4s(9)  ==
  settings: updateMethod=DISCRETE
  data: I input; Gate output size=3; FEM input size=2; iAref input; iBref input; mode input; jo output

function [Gate,jo]       = fcn(I,FEM,iAref,iBref,mode)
%function Gate       = fcn(I,FEM,iAref,iBref,mode,Ts, R, Ls, ud, gmax,dyV, Tab)


%%%%%Init Parameters%%%%%%%

Ts=single(3e-5);
R=single(1.1) ;
%Ls=single(0.002871);
Ls=single(0.00372);
ud=single(170);
gmax=single(1000);
n=single(9);

% Div=single(4); %%%%Numero de divisiones 
% dy0=single(0.12);
dyV=single(0.85);


%Tp=single(Ts*0.9);
 persistent    Gop jop Gates 
     if isempty(Gates)
        Gates=single([0,0,0]');
        Gop=gmax;
        jop=single(1);
  
     end


%%%%%%Read mesurments%%%%%%%%%%%%
iA=I(1);
iB=I(2);
eA=-FEM(1);
eB=-FEM(2);
moder=mode;

% % 
% % indexv=[1,1,1,1,1,1,1,1,1,1,2,2,2,2,3;
% %         1,1,1,1,1,1,2,2,2,3,2,2,2,3,3;
% %         1,1,1,2,2,3,2,2,3,3,2,2,3,3,3;
% %         1,2,3,2,3,3,2,3,3,3,2,3,3,3,3;];

Tab=single([0.25	0;
0	0.25;
0.5	0;
0	0.5;
0.75	0;
0	0.75;
1	0;
0	1;
0	0]);

if mode==1
   u1=ud*[0	,	0	;
2/3	,	0	;
1/3	,	1/sqrt(3)];
elseif mode==2
   u1=ud*[0	,	0	;
1/3	,	1/sqrt(3)	;
-1/3	,	1/sqrt(3)	;];   
elseif mode==3
   u1=ud*[0	,	0	;
-1/3	,	1/sqrt(3)	;
-2/3	,	0	;];  
 elseif mode==4
   u1=ud*[0	,	0	;
-2/3	,	0	;
-1/3	,	-1/sqrt(3)	;];
 elseif mode==5
   u1=ud*[0	,	0	;
-1/3	,	-1/sqrt(3)	;
1/3	,	-1/sqrt(3)	;];
 elseif mode==6
  u1=ud*[0	,	0	;
1/3	,	-1/sqrt(3)	;
2/3	,	0	;];
else
  u1=ud*[0	,	0	;
2/3	,	0	;
1/3	,	1/sqrt(3)]; 
end

%%%%%%%%FSMPC%%%%%%%%%%%%%%%%%%%%%%%%%%%%%%%%%%%%%

     Gop=gmax;
     jop=single(1);
     uA1=u1(2,1);
     uB1=u1(2,2);
     uA2=u1(3,1);
     uB2=u1(3,2);

%%%%%%For n loop  %%%%%% 
     for j= 1:n    
   
    T1=Tab(j,1);
    T2=Tab(j,2);
    uA=dyV*(T1*uA1 + T2*uA2);%+dy0*uAnull;
    uB=dyV*(T1*uB1 + T2*uB2);%+dy0*uAnull;

%%%%%%For loop 3 combinacion de vectores%%%%%% 

     iA1= iA + (1/Ls)*(Ts*uA)- (Ts/Ls)*(eA+R*iA);
     iB1=iB + (1/Ls)*(Ts*uB)- (Ts/Ls)*(eB+R*iB);
     
     G=(iAref-iA1)^2+(iBref-iB1)^2 ; 

          if G<Gop
          Gop=G;
          jop=j;
          
          end
     end
%%%%Apply conmutation states%%%%%%%%%%%%%%%%%%%%%%%  
Ta=dyV*Tab(jop,1);
Tb=dyV*Tab(jop,2);
To=1-Ta-Tb-0.15;

% TA=(moder==1)*(Tb+Ta)+(moder==6)*(Tb+Ta)+(moder==2)*(Ta)+(moder==5)*(Tb);
% TB=(moder==1)*(Tb)+(moder==2)*(Tb+Ta)+(moder==3)*(Tb+Ta)+(moder==4)*(Ta);
% TC=(moder==6)*(Ta)+(moder==3)*(Tb)+(moder==4)*(Tb+Ta)+(moder==5)*(Tb+Ta);
% 
TA=(mode==1)*(To+Tb+Ta)+(mode==6)*(To+Tb+Ta)+(mode==2)*(To+Ta)+(mode==3)*(To)+(mode==4)*(To)+(mode==5)*(To+Tb);
TB=(mode==6)*(To)+(mode==1)*(To+Tb)+(mode==2)*(To+Tb+Ta)+(mode==3)*(To+Tb+Ta)+(mode==4)*(To+Ta)+(mode==5)*(To);
TC=(mode==6)*(To+Ta)+(mode==1)*(To)+(mode==2)*(To)+(mode==3)*(To+Tb)+(mode==4)*(To+Tb+Ta)+(mode==5)*(To+Tb+Ta);
% 

Gates=[TA,TB,TC]';
Gate=Gates;
jo=jop;

== matlab function MicroFSMPCCLACPU1/ADC-PWM /Control_System/CLA Subsystem Current control/FS-MPC1_ CLA 10s(21) ==
  settings: updateMethod=DISCRETE
  data: I input; Gate output size=3; FEM input size=2; iAref input; iBref input; mode input; jo output

function [Gate,jo]       = fcn(I,FEM,iAref,iBref,mode)
%function Gate       = fcn(I,FEM,iAref,iBref,mode,Ts, R, Ls, ud, gmax,dyV, Tab)


%%%%%Init Parameters%%%%%%%

Ts=single(3e-5);
R=single(1.1) ;
%Ls=single(0.002871);
Ls=single(0.00372);
ud=single(170);
gmax=single(1000);
n=single(21);

% Div=single(4); %%%%Numero de divisiones 
% dy0=single(0.12);
dyV=single(0.85);


%Tp=single(Ts*0.9);
 persistent    Gop jop Gates 
     if isempty(Gates)
        Gates=single([0,0,0]');
        Gop=gmax;
        jop=single(1);
  
     end


%%%%%%Read mesurments%%%%%%%%%%%%
iA=I(1);
iB=I(2);
eA=-FEM(1);
eB=-FEM(2);
moder=mode;

% % 
% % indexv=[1,1,1,1,1,1,1,1,1,1,2,2,2,2,3;
% %         1,1,1,1,1,1,2,2,2,3,2,2,2,3,3;
% %         1,1,1,2,2,3,2,2,3,3,2,2,3,3,3;
% %         1,2,3,2,3,3,2,3,3,3,2,3,3,3,3;];

Tab=single([0.10	0;
0	0.10;
0.20	0;
0	0.20;
0.30	0;
0	0.3;
0.40	0;
0	0.4;
0.5	0;
0	0.5;
0.6	0;
0	0.6;
0.7	0;
0	0.7;
0.8	0;
0	0.8;
0.9	0;
0	0.9;
1	0;
0	1;
0	0]);

if mode==1
   u1=ud*[0	,	0	;
2/3	,	0	;
1/3	,	1/sqrt(3)];
elseif mode==2
   u1=ud*[0	,	0	;
1/3	,	1/sqrt(3)	;
-1/3	,	1/sqrt(3)	;];   
elseif mode==3
   u1=ud*[0	,	0	;
-1/3	,	1/sqrt(3)	;
-2/3	,	0	;];  
 elseif mode==4
   u1=ud*[0	,	0	;
-2/3	,	0	;
-1/3	,	-1/sqrt(3)	;];
 elseif mode==5
   u1=ud*[0	,	0	;
-1/3	,	-1/sqrt(3)	;
1/3	,	-1/sqrt(3)	;];
 elseif mode==6
  u1=ud*[0	,	0	;
1/3	,	-1/sqrt(3)	;
2/3	,	0	;];
else
  u1=ud*[0	,	0	;
2/3	,	0	;
1/3	,	1/sqrt(3)]; 
end

%%%%%%%%FSMPC%%%%%%%%%%%%%%%%%%%%%%%%%%%%%%%%%%%%%

     Gop=gmax;
     jop=single(1);
     uA1=u1(2,1);
     uB1=u1(2,2);
     uA2=u1(3,1);
     uB2=u1(3,2);

%%%%%%For n loop  %%%%%% 
     for j= 1:n    
   
    T1=Tab(j,1);
    T2=Tab(j,2);
    uA=dyV*(T1*uA1 + T2*uA2);%+dy0*uAnull;
    uB=dyV*(T1*uB1 + T2*uB2);%+dy0*uAnull;

%%%%%%For loop 3 combinacion de vectores%%%%%% 

     iA1= iA + (1/Ls)*(Ts*uA)- (Ts/Ls)*(eA+R*iA);
     iB1=iB + (1/Ls)*(Ts*uB)- (Ts/Ls)*(eB+R*iB);
     
     G=(iAref-iA1)^2+(iBref-iB1)^2 ; 

          if G<Gop
          Gop=G;
          jop=j;
          
          end
     end
%%%%Apply conmutation states%%%%%%%%%%%%%%%%%%%%%%%  
Ta=dyV*Tab(jop,1);
Tb=dyV*Tab(jop,2);
To=1-Ta-Tb-0.15;

% TA=(moder==1)*(Tb+Ta)+(moder==6)*(Tb+Ta)+(moder==2)*(Ta)+(moder==5)*(Tb);
% TB=(moder==1)*(Tb)+(moder==2)*(Tb+Ta)+(moder==3)*(Tb+Ta)+(moder==4)*(Ta);
% TC=(moder==6)*(Ta)+(moder==3)*(Tb)+(moder==4)*(Tb+Ta)+(moder==5)*(Tb+Ta);
% 
TA=(mode==1)*(To+Tb+Ta)+(mode==6)*(To+Tb+Ta)+(mode==2)*(To+Ta)+(mode==3)*(To)+(mode==4)*(To)+(mode==5)*(To+Tb);
TB=(mode==6)*(To)+(mode==1)*(To+Tb)+(mode==2)*(To+Tb+Ta)+(mode==3)*(To+Tb+Ta)+(mode==4)*(To+Ta)+(mode==5)*(To);
TC=(mode==6)*(To+Ta)+(mode==1)*(To)+(mode==2)*(To)+(mode==3)*(To+Tb)+(mode==4)*(To+Tb+Ta)+(mode==5)*(To+Tb+Ta);
% 

Gates=[TA,TB,TC]';
Gate=Gates;
jo=jop;

== matlab function MicroFSMPCCLACPU1/ADC-PWM /Control_System/CLA Subsystem Current control/FS-MPC1_ CLA 7s(15)  ==
  settings: updateMethod=DISCRETE
  data: I input; Gate output size=3; FEM input size=2; iAref input; iBref input; mode input; ud input

function Gate        = fcn(I,FEM,iAref,iBref,mode,ud)
%function Gate       = fcn(I,FEM,iAref,iBref,mode,Ts, R, Ls, ud, gmax,dyV, Tab)


%%%%%Init Parameters%%%%%%%

Ts=single(3e-5);
R=single(1.1) ;
%Ls=single(0.002871);
Ls=single(0.00372);
%ud=single(170);
gmax=single(1000);
n=single(15);

% Div=single(4); %%%%Numero de divisiones 
% dy0=single(0.12);
dyV=single(0.85);


%Tp=single(Ts*0.9);
 persistent    Gop jop Gates 
     if isempty(Gates)
        Gates=single([0,0,0]');
        Gop=gmax;
        jop=single(1);
  
     end


%%%%%%Read mesurments%%%%%%%%%%%%
iA=I(1);
iB=I(2);
eA=-FEM(1);
eB=-FEM(2);
moder=mode;

% % 
% % indexv=[1,1,1,1,1,1,1,1,1,1,2,2,2,2,3;
% %         1,1,1,1,1,1,2,2,2,3,2,2,2,3,3;
% %         1,1,1,2,2,3,2,2,3,3,2,2,3,3,3;
% %         1,2,3,2,3,3,2,3,3,3,2,3,3,3,3;];

Tab=single([0.143	0;
0	0.143;
0.286	0;
0	0.286;
0.429	0;
0	0.429;
0.572	0;
0	0.572;
0.715	0;
0	0.715;
0.858	0;
0	0.858;
1	0;
0	1;
0	0]);

if mode==1
   u1=ud*[0	,	0	;
2/3	,	0	;
1/3	,	1/sqrt(3)];
elseif mode==2
   u1=ud*[0	,	0	;
1/3	,	1/sqrt(3)	;
-1/3	,	1/sqrt(3)	;];   
elseif mode==3
   u1=ud*[0	,	0	;
-1/3	,	1/sqrt(3)	;
-2/3	,	0	;];  
 elseif mode==4
   u1=ud*[0	,	0	;
-2/3	,	0	;
-1/3	,	-1/sqrt(3)	;];
 elseif mode==5
   u1=ud*[0	,	0	;
-1/3	,	-1/sqrt(3)	;
1/3	,	-1/sqrt(3)	;];
 elseif mode==6
  u1=ud*[0	,	0	;
1/3	,	-1/sqrt(3)	;
2/3	,	0	;];
else
  u1=ud*[0	,	0	;
2/3	,	0	;
1/3	,	1/sqrt(3)]; 
end

%%%%%%%%FSMPC%%%%%%%%%%%%%%%%%%%%%%%%%%%%%%%%%%%%%

     Gop=gmax;
     jop=single(1);
     uA1=u1(2,1);
     uB1=u1(2,2);
     uA2=u1(3,1);
     uB2=u1(3,2);

%%%%%%For n loop  %%%%%% 
     for j= 1:n    
   
    T1=Tab(j,1);
    T2=Tab(j,2);
    uA=dyV*(T1*uA1 + T2*uA2);%+dy0*uAnull;
    uB=dyV*(T1*uB1 + T2*uB2);%+dy0*uAnull;

%%%%%%For loop 3 combinacion de vectores%%%%%% 

     iA1= iA + (1/Ls)*(Ts*uA)- (Ts/Ls)*(eA+R*iA);
     iB1=iB + (1/Ls)*(Ts*uB)- (Ts/Ls)*(eB+R*iB);
     
     G=(iAref-iA1)^2+(iBref-iB1)^2 ; 

          if G<Gop
          Gop=G;
          jop=j;
          
          end
     end
%%%%Apply conmutation states%%%%%%%%%%%%%%%%%%%%%%%  
Ta=dyV*Tab(jop,1);
Tb=dyV*Tab(jop,2);
To=1-Ta-Tb-0.15;

% TA=(moder==1)*(Tb+Ta)+(moder==6)*(Tb+Ta)+(moder==2)*(Ta)+(moder==5)*(Tb);
% TB=(moder==1)*(Tb)+(moder==2)*(Tb+Ta)+(moder==3)*(Tb+Ta)+(moder==4)*(Ta);
% TC=(moder==6)*(Ta)+(moder==3)*(Tb)+(moder==4)*(Tb+Ta)+(moder==5)*(Tb+Ta);
% 
TA=(mode==1)*(To+Tb+Ta)+(mode==6)*(To+Tb+Ta)+(mode==2)*(To+Ta)+(mode==3)*(To)+(mode==4)*(To)+(mode==5)*(To+Tb);
TB=(mode==6)*(To)+(mode==1)*(To+Tb)+(mode==2)*(To+Tb+Ta)+(mode==3)*(To+Tb+Ta)+(mode==4)*(To+Ta)+(mode==5)*(To);
TC=(mode==6)*(To+Ta)+(mode==1)*(To)+(mode==2)*(To)+(mode==3)*(To+Tb)+(mode==4)*(To+Tb+Ta)+(mode==5)*(To+Tb+Ta);
% 

Gates=[TA,TB,TC]';
Gate=Gates;
%jo=jop;
